simulink library "EntertainmentLevelDetectorBtc"  (R2022b)
settings: Solver=VariableStepAuto  StartTime=0.0  StopTime=10.0  RelTol=1e-3
libraries: TuneVar x25, LevelDetectorLibraryLib x4, PoolIirBtc x2, PooliirLib x2, HandyTextFile x1
settings Model: Creator=kl13806  LastModifiedBy=kl13806
settings SolverCC: AlgebraicLoopSolver=TrustRegion
settings DebuggingCC: UnconnectedInputMsg=warning  UnconnectedOutputMsg=warning  UnconnectedLineMsg=warning  SFMachineParentedDataDiag=warning
settings ModelReferenceCC: EnableRefExpFcnMdlSchedulingChecks=on
settings RTWCC: DLArmComputeVersion=19.05

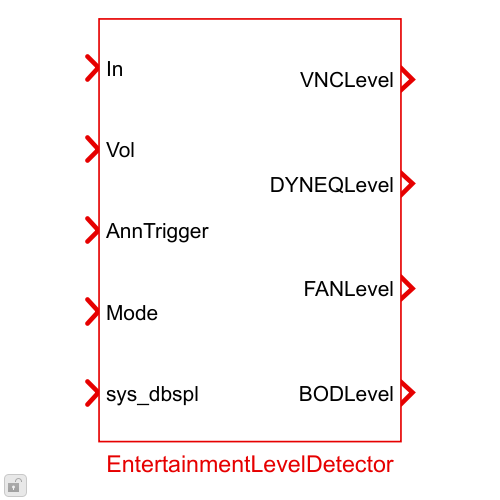
[thumbnail: Simulink's stored preview of the top-level diagram]
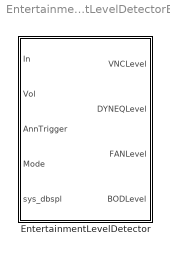
== system EntertainmentLevelDetectorBtc ==
  EntertainmentLevelDetector : Subsystem  mask(Level Detector for VNC, Dyanmic EQ, Fan and Boost-on-Demand){Config=[]}
      mask prompts: Config "EntertainmentLevelDetectorConfig"
      mask help: Level detector of entertainment audio in Audio Pilot.
      mask init:
      | blkh=gcbh;
      | Config=BTConfig.Assert(blkh,Config);
      | 
      | Config.Validate();

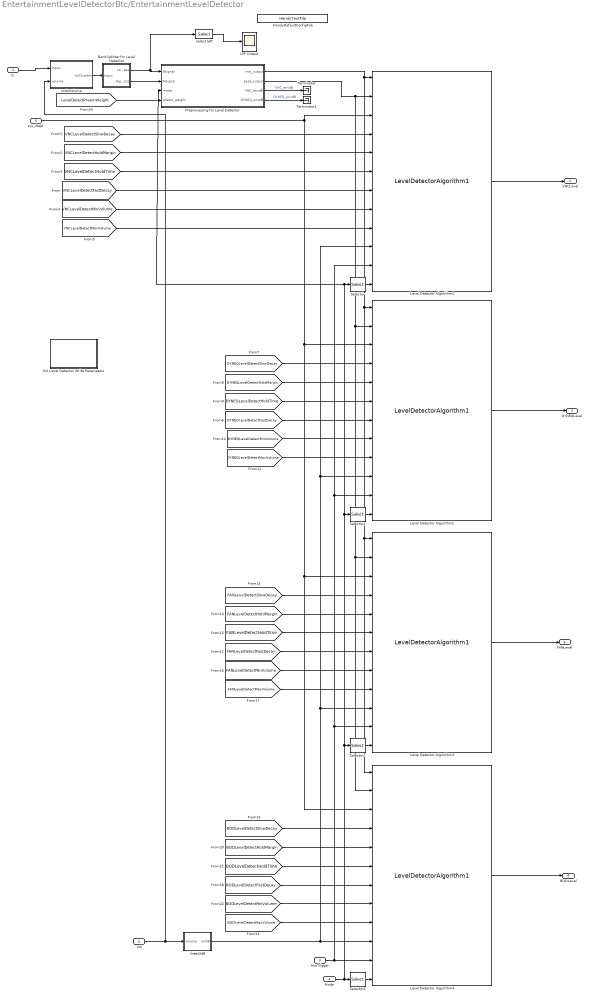
== system EntertainmentLevelDetectorBtc/EntertainmentLevelDetector ==
  In : Inport
  Vol : Inport  Port=2
  AnnTrigger : Inport  Port=3
  Mode : Inport  Port=4
  sys_dbspl : Inport  Port=5
  Band Splitter for Level Detector : Subsystem
  Ent Level Detector Write Parameters : Subsystem
  HandyDefaultConfigFile : HandyTextFile/HandyTextFile  TemplateSource=Config  FileSuffix=Init  OpenDialogOnLoad=off  UseThisBlockName=off  AddGrandParentNamePrefix=off  TheDefaultText=|  ShowInLibBrowser=on
      | % $(FILENAME) Setup model parameters for each "Init" callback (e.g. update diagram)
      | sample_rate_in_hertz = 44100;
      | frame_size = 32;
      | sysin_channel_count = 2;
      settings: SourceProductName=Bose Talaria
  LPF Output : Scope
  Level Detector Algorithm{1..4} (4 alike) : LevelDetectorLibraryLib/LevelDetectorAlgorithm1  Fd=Config.DlgDecRate
  Preprocessing for Level Detector : MATLAB Function  TreatAsAtomicUnit=on
  Selector : Selector  InputPortWidth=4  IndexOptions=Index vector (dialog)  Indices=[1]  OutputSizes=1
  Selector1 : Selector  InputPortWidth=4  IndexOptions=Index vector (dialog)  Indices=[2]  OutputSizes=1
  Selector2 : Selector  InputPortWidth=4  IndexOptions=Index vector (dialog)  Indices=[3]  OutputSizes=1
  Selector3 : Selector  InputPortWidth=4  IndexOptions=Index vector (dialog)  Indices=[4]  OutputSizes=1
  Terminator : Terminator
  Terminator1 : Terminator
  linear2dB : MATLAB Function  TreatAsAtomicUnit=on
  select left : Selector  NumberOfDimensions=2  InputPortWidth=3  IndexOptions=Select all,Index vector (dialog)  Indices=[1 3],1  OutputSizes=1,1
  undoVolume : MATLAB Function  TreatAsAtomicUnit=on
  VNCLevel : Outport  VectorParamsAs1DForOutWhenUnconnected=off
  DYNEQLevel : Outport  Port=2  VectorParamsAs1DForOutWhenUnconnected=off
  FANLevel : Outport  Port=3  VectorParamsAs1DForOutWhenUnconnected=off
  BODLevel : Outport  Port=4  VectorParamsAs1DForOutWhenUnconnected=off
  wires:
  In/1 -> undoVolume/1(input)
  undoVolume/1(fullScaleIn) -> Band Splitter for Level Detector/1(Input)
  [LevelDetectPreemWeight] -> Preprocessing for Level Detector/4(preem_weight)
  Preprocessing for Level Detector/4(DYNEQ_envdB) -> Terminator1/1  "DYNEQ_envdB"
  Preprocessing for Level Detector/3(VNC_envdB) -> Terminator/1  "VNC_envdB"
  [BODLevelDetectHoldMargin] -> Level Detector Algorithm4/5
  [BODLevelDetectHoldTime] -> Level Detector Algorithm4/6
  [BODLevelDetectSlowDecay] -> Level Detector Algorithm4/4
  [BODLevelDetectFastDecay] -> Level Detector Algorithm4/7
  Selector3/1 -> Level Detector Algorithm4/12
  Selector2/1 -> Level Detector Algorithm3/12
  Selector1/1 -> Level Detector Algorithm2/12
  Selector/1 -> Level Detector Algorithm1/12
  Mode/1 -> Selector/1, Preprocessing for Level Detector/3(mode), Selector1/1, Selector2/1, Selector3/1
  Level Detector Algorithm1/1 -> VNCLevel/1
  linear2dB/1(voldB) -> Level Detector Algorithm1/10, Level Detector Algorithm2/10, Level Detector Algorithm3/10, Level Detector Algorithm4/10
  sys_dbspl/1 -> Level Detector Algorithm1/3, Level Detector Algorithm3/3, Level Detector Algorithm4/3, Level Detector Algorithm2/3
  [VNCLevelDetectMaxVolume] -> Level Detector Algorithm1/9
  [BODLevelDetectMaxVolume] -> Level Detector Algorithm4/9
  [BODLevelDetectMinVolume] -> Level Detector Algorithm4/8
  Level Detector Algorithm4/1 -> BODLevel/1
  Preprocessing for Level Detector/2(peak_output) -> Level Detector Algorithm3/2, Level Detector Algorithm4/2, Level Detector Algorithm2/2, Level Detector Algorithm1/2
  [VNCLevelDetectMinVolume] -> Level Detector Algorithm1/8
  [VNCLevelDetectFastDecay] -> Level Detector Algorithm1/7
  [VNCLevelDetectHoldTime] -> Level Detector Algorithm1/6
  [VNCLevelDetectHoldMargin] -> Level Detector Algorithm1/5
  [VNCLevelDetectSlowDecay] -> Level Detector Algorithm1/4
  Vol/1 -> linear2dB/1(volume), undoVolume/2(volume)
  AnnTrigger/1 -> Level Detector Algorithm1/11, Level Detector Algorithm2/11, Level Detector Algorithm3/11, Level Detector Algorithm4/11
  select left/1 -> LPF Output/1
  [DYNEQLevelDetectSlowDecay] -> Level Detector Algorithm2/4
  [DYNEQLevelDetectHoldMargin] -> Level Detector Algorithm2/5
  [DYNEQLevelDetectHoldTime] -> Level Detector Algorithm2/6
  [DYNEQLevelDetectFastDecay] -> Level Detector Algorithm2/7
  [DYNEQLevelDetectMinVolume] -> Level Detector Algorithm2/8
  [DYNEQLevelDetectMaxVolume] -> Level Detector Algorithm2/9
  [FANLevelDetectSlowDecay] -> Level Detector Algorithm3/4
  [FANLevelDetectHoldMargin] -> Level Detector Algorithm3/5
  [FANLevelDetectHoldTime] -> Level Detector Algorithm3/6
  [FANLevelDetectFastDecay] -> Level Detector Algorithm3/7
  [FANLevelDetectMinVolume] -> Level Detector Algorithm3/8
  [FANLevelDetectMaxVolume] -> Level Detector Algorithm3/9
  Preprocessing for Level Detector/1(rms_output) -> Level Detector Algorithm3/1, Level Detector Algorithm4/1, Level Detector Algorithm2/1, Level Detector Algorithm1/1
  Band Splitter for Level Detector/1(LowPass) -> select left/1, Preprocessing for Level Detector/1(Bsignal)
  Band Splitter for Level Detector/2(HighPass) -> Preprocessing for Level Detector/2(Msignal)
  Level Detector Algorithm2/1 -> DYNEQLevel/1
  Level Detector Algorithm3/1 -> FANLevel/1

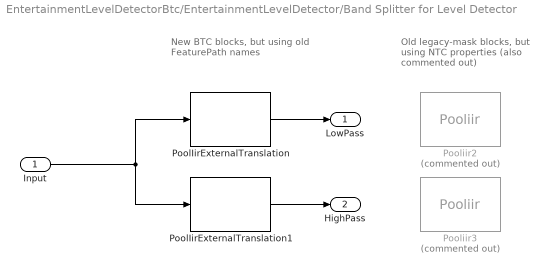
== system EntertainmentLevelDetectorBtc/EntertainmentLevelDetector/Band Splitter for Level Detector ==
  note: Old legacy-mask blocks,
      | but using NTC properties
      | (also commented out)
  note: New BTC blocks, but using
      | old FeaturePath names
  Input : Inport
  PoolIirExternalTranslation : PoolIirBtc/PoolIirExternalTranslation  Config=Config.level_detect_preemphasis_lpf_  FeatureName=level_detect_preemphasis_lpf_
      settings: SourceProductName=Bose Blocklib
  PoolIirExternalTranslation1 : PoolIirBtc/PoolIirExternalTranslation  Config=Config.level_detect_preemphasis_hpf_  FeatureName=level_detect_preemphasis_hpf_
      settings: SourceProductName=Bose Blocklib
  Pooliir2 : PooliirLib/Pooliir  Commented=on  maxNumStages=Config.DlgBsMaxNumStages  numStages=Config.DlgBsNumStages  coeffs=Config.DlgBsLpCoeffs  FeatureName=level_detect_preemphasis_lpf_
  Pooliir3 : PooliirLib/Pooliir  Commented=on  maxNumStages=Config.DlgBsMaxNumStages  numStages=Config.DlgBsNumStages  coeffs=Config.DlgBsHpCoeffs  FeatureName=level_detect_preemphasis_hpf_
  LowPass : Outport  VectorParamsAs1DForOutWhenUnconnected=off
  HighPass : Outport  Port=2  VectorParamsAs1DForOutWhenUnconnected=off
  wires:
  Input/1 -> PoolIirExternalTranslation1/1, PoolIirExternalTranslation/1
  PoolIirExternalTranslation/1 -> LowPass/1
  PoolIirExternalTranslation1/1 -> HighPass/1

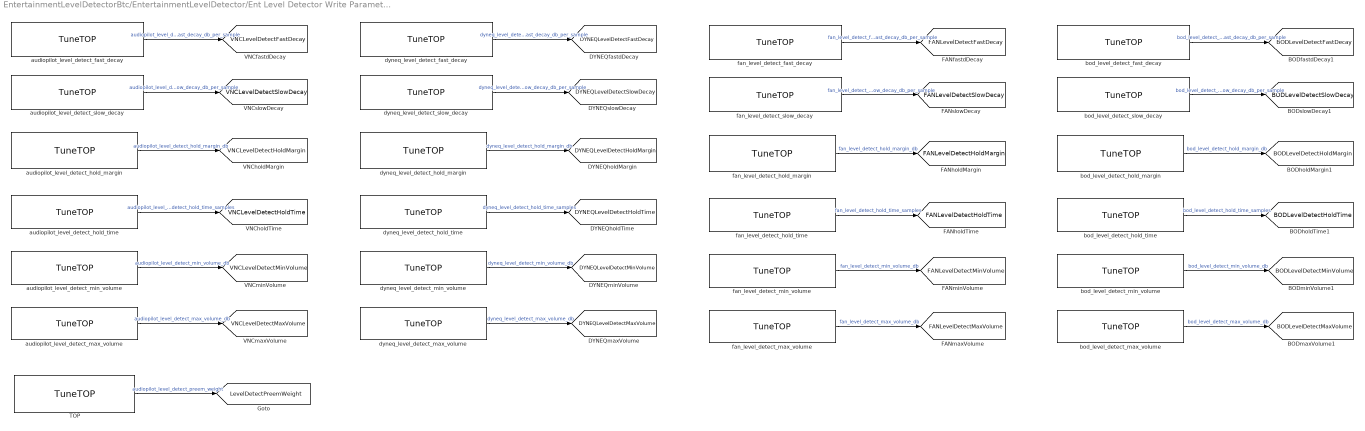
== system EntertainmentLevelDetectorBtc/EntertainmentLevelDetector/Ent Level Detector Write Parameters ==
  TOP : TuneVar/TuneTOP  TriggerInit=[-285 479 -80 541]  TopName=audiopilot_level_detect_preem_weight  TuneName=audiopilot_level_detect_preem_weight  DataType=Inherit: Same as input  TunabilityNumber=1  MinValue=[]  MaxValue=[]  BankNumber=0  PreOverlay=false  PostOverlay=false  UseSameName=on  MaskValue=single(4.0)
      settings: SourceProductName=Bose Talaria
  audiopilot_level_detect_fast_decay : TuneVar/TuneTOP  TriggerInit=[-290 -124 -65 -66]  TopName=audiopilot_level_detect_fast_decay_db_per_sample  TuneName=audiopilot_level_detect_fast_decay_db_per_sample  DataType=Inherit: Same as input  TunabilityNumber=1  MinValue=[]  MaxValue=[]  BankNumber=0  PreOverlay=false  PostOverlay=false  UseSameName=on  MaskValue=Config.DlgFastDecay
      settings: SourceProductName=Bose Talaria
  audiopilot_level_detect_hold_margin : TuneVar/TuneTOP  TriggerInit=[-290 64 -75 126]  TopName=audiopilot_level_detect_hold_margin_db  TuneName=audiopilot_level_detect_hold_margin_db  DataType=Inherit: Same as input  TunabilityNumber=1  MinValue=[]  MaxValue=[]  BankNumber=0  PreOverlay=false  PostOverlay=false  UseSameName=on  MaskValue=Config.DefaultHoldMargin
      settings: SourceProductName=Bose Talaria
  audiopilot_level_detect_hold_time : TuneVar/TuneTOP  TriggerInit=[-290 172 -75 228]  TopName=audiopilot_level_detect_hold_time_samples  TuneName=audiopilot_level_detect_hold_time_samples  DataType=Inherit: Same as input  TunabilityNumber=1  MinValue=[]  MaxValue=[]  BankNumber=0  PreOverlay=false  PostOverlay=false  UseSameName=on  MaskValue=Config.DlgHoldTime
      settings: SourceProductName=Bose Talaria
  audiopilot_level_detect_max_volume : TuneVar/TuneTOP  TriggerInit=[-290 362 -75 418]  TopName=audiopilot_level_detect_max_volume_db  TuneName=audiopilot_level_detect_max_volume_db  DataType=Inherit: Same as input  TunabilityNumber=1  MinValue=[]  MaxValue=[]  BankNumber=0  PreOverlay=false  PostOverlay=false  UseSameName=on  MaskValue=Config.DefaultMaxVolDbSpl
      settings: SourceProductName=Bose Talaria
  audiopilot_level_detect_min_volume : TuneVar/TuneTOP  TriggerInit=[-290 267 -75 323]  TopName=audiopilot_level_detect_min_volume_db  TuneName=audiopilot_level_detect_min_volume_db  DataType=Inherit: Same as input  TunabilityNumber=1  MinValue=[]  MaxValue=[]  BankNumber=0  PreOverlay=false  PostOverlay=false  UseSameName=on  MaskValue=Config.DefaultMinVolDpSpl
      settings: SourceProductName=Bose Talaria
  audiopilot_level_detect_slow_decay : TuneVar/TuneTOP  TriggerInit=[-290 -34 -65 24]  TopName=audiopilot_level_detect_slow_decay_db_per_sample  TuneName=audiopilot_level_detect_slow_decay_db_per_sample  DataType=Inherit: Same as input  TunabilityNumber=1  MinValue=[]  MaxValue=[]  BankNumber=0  PreOverlay=false  PostOverlay=false  UseSameName=on  MaskValue=Config.DlgSlowDecay
      settings: SourceProductName=Bose Talaria
  bod_level_detect_fast_decay : TuneVar/TuneTOP  TriggerInit=[1495 -119 1720 -61]  TopName=bod_level_detect_fast_decay_db_per_sample  TuneName=bod_level_detect_fast_decay_db_per_sample  DataType=Inherit: Same as input  TunabilityNumber=1  MinValue=[]  MaxValue=[]  BankNumber=0  PreOverlay=false  PostOverlay=false  UseSameName=on  MaskValue=Config.DlgFastDecay
      settings: SourceProductName=Bose Talaria
  bod_level_detect_hold_margin : TuneVar/TuneTOP  TriggerInit=[1495 69 1710 131]  TopName=bod_level_detect_hold_margin_db  TuneName=bod_level_detect_hold_margin_db  DataType=Inherit: Same as input  TunabilityNumber=1  MinValue=[]  MaxValue=[]  BankNumber=0  PreOverlay=false  PostOverlay=false  UseSameName=on  MaskValue=Config.DefaultHoldMargin
      settings: SourceProductName=Bose Talaria
  bod_level_detect_hold_time : TuneVar/TuneTOP  TriggerInit=[1495 177 1710 233]  TopName=bod_level_detect_hold_time_samples  TuneName=bod_level_detect_hold_time_samples  DataType=Inherit: Same as input  TunabilityNumber=1  MinValue=[]  MaxValue=[]  BankNumber=0  PreOverlay=false  PostOverlay=false  UseSameName=on  MaskValue=Config.DlgHoldTime
      settings: SourceProductName=Bose Talaria
  bod_level_detect_max_volume : TuneVar/TuneTOP  TriggerInit=[1495 367 1710 423]  TopName=bod_level_detect_max_volume_db  TuneName=bod_level_detect_max_volume_db  DataType=Inherit: Same as input  TunabilityNumber=1  MinValue=[]  MaxValue=[]  BankNumber=0  PreOverlay=false  PostOverlay=false  UseSameName=on  MaskValue=Config.DefaultMaxVolDbSpl
      settings: SourceProductName=Bose Talaria
  bod_level_detect_min_volume : TuneVar/TuneTOP  TriggerInit=[1495 272 1710 328]  TopName=bod_level_detect_min_volume_db  TuneName=bod_level_detect_min_volume_db  DataType=Inherit: Same as input  TunabilityNumber=1  MinValue=[]  MaxValue=[]  BankNumber=0  PreOverlay=false  PostOverlay=false  UseSameName=on  MaskValue=Config.DefaultMinVolDpSpl
      settings: SourceProductName=Bose Talaria
  bod_level_detect_slow_decay : TuneVar/TuneTOP  TriggerInit=[1495 -29 1720 29]  TopName=bod_level_detect_slow_decay_db_per_sample  TuneName=bod_level_detect_slow_decay_db_per_sample  DataType=Inherit: Same as input  TunabilityNumber=1  MinValue=[]  MaxValue=[]  BankNumber=0  PreOverlay=false  PostOverlay=false  UseSameName=on  MaskValue=Config.DlgSlowDecay
      settings: SourceProductName=Bose Talaria
  dyneq_level_detect_fast_decay : TuneVar/TuneTOP  TriggerInit=[305 -124 530 -66]  TopName=dyneq_level_detect_fast_decay_db_per_sample  TuneName=dyneq_level_detect_fast_decay_db_per_sample  DataType=Inherit: Same as input  TunabilityNumber=1  MinValue=[]  MaxValue=[]  BankNumber=0  PreOverlay=false  PostOverlay=false  UseSameName=on  MaskValue=Config.DlgFastDecay
      settings: SourceProductName=Bose Talaria
  dyneq_level_detect_hold_margin : TuneVar/TuneTOP  TriggerInit=[305 64 520 126]  TopName=dyneq_level_detect_hold_margin_db  TuneName=dyneq_level_detect_hold_margin_db  DataType=Inherit: Same as input  TunabilityNumber=1  MinValue=[]  MaxValue=[]  BankNumber=0  PreOverlay=false  PostOverlay=false  UseSameName=on  MaskValue=Config.DefaultHoldMargin
      settings: SourceProductName=Bose Talaria
  dyneq_level_detect_hold_time : TuneVar/TuneTOP  TriggerInit=[305 172 520 228]  TopName=dyneq_level_detect_hold_time_samples  TuneName=dyneq_level_detect_hold_time_samples  DataType=Inherit: Same as input  TunabilityNumber=1  MinValue=[]  MaxValue=[]  BankNumber=0  PreOverlay=false  PostOverlay=false  UseSameName=on  MaskValue=Config.DlgHoldTime
      settings: SourceProductName=Bose Talaria
  dyneq_level_detect_max_volume : TuneVar/TuneTOP  TriggerInit=[305 362 520 418]  TopName=dyneq_level_detect_max_volume_db  TuneName=dyneq_level_detect_max_volume_db  DataType=Inherit: Same as input  TunabilityNumber=1  MinValue=[]  MaxValue=[]  BankNumber=0  PreOverlay=false  PostOverlay=false  UseSameName=on  MaskValue=Config.DefaultMaxVolDbSpl
      settings: SourceProductName=Bose Talaria
  dyneq_level_detect_min_volume : TuneVar/TuneTOP  TriggerInit=[305 267 520 323]  TopName=dyneq_level_detect_min_volume_db  TuneName=dyneq_level_detect_min_volume_db  DataType=Inherit: Same as input  TunabilityNumber=1  MinValue=[]  MaxValue=[]  BankNumber=0  PreOverlay=false  PostOverlay=false  UseSameName=on  MaskValue=Config.DefaultMinVolDpSpl
      settings: SourceProductName=Bose Talaria
  dyneq_level_detect_slow_decay : TuneVar/TuneTOP  TriggerInit=[305 -34 530 24]  TopName=dyneq_level_detect_slow_decay_db_per_sample  TuneName=dyneq_level_detect_slow_decay_db_per_sample  DataType=Inherit: Same as input  TunabilityNumber=1  MinValue=[]  MaxValue=[]  BankNumber=0  PreOverlay=false  PostOverlay=false  UseSameName=on  MaskValue=Config.DlgSlowDecay
      settings: SourceProductName=Bose Talaria
  fan_level_detect_fast_decay : TuneVar/TuneTOP  TriggerInit=[900 -119 1125 -61]  TopName=fan_level_detect_fast_decay_db_per_sample  TuneName=fan_level_detect_fast_decay_db_per_sample  DataType=Inherit: Same as input  TunabilityNumber=1  MinValue=[]  MaxValue=[]  BankNumber=0  PreOverlay=false  PostOverlay=false  UseSameName=on  MaskValue=Config.DlgFastDecay
      settings: SourceProductName=Bose Talaria
  fan_level_detect_hold_margin : TuneVar/TuneTOP  TriggerInit=[900 69 1115 131]  TopName=fan_level_detect_hold_margin_db  TuneName=fan_level_detect_hold_margin_db  DataType=Inherit: Same as input  TunabilityNumber=1  MinValue=[]  MaxValue=[]  BankNumber=0  PreOverlay=false  PostOverlay=false  UseSameName=on  MaskValue=Config.DefaultHoldMargin
      settings: SourceProductName=Bose Talaria
  fan_level_detect_hold_time : TuneVar/TuneTOP  TriggerInit=[900 177 1115 233]  TopName=fan_level_detect_hold_time_samples  TuneName=fan_level_detect_hold_time_samples  DataType=Inherit: Same as input  TunabilityNumber=1  MinValue=[]  MaxValue=[]  BankNumber=0  PreOverlay=false  PostOverlay=false  UseSameName=on  MaskValue=Config.DlgHoldTime
      settings: SourceProductName=Bose Talaria
  fan_level_detect_max_volume : TuneVar/TuneTOP  TriggerInit=[900 367 1115 423]  TopName=fan_level_detect_max_volume_db  TuneName=fan_level_detect_max_volume_db  DataType=Inherit: Same as input  TunabilityNumber=1  MinValue=[]  MaxValue=[]  BankNumber=0  PreOverlay=false  PostOverlay=false  UseSameName=on  MaskValue=Config.DefaultMaxVolDbSpl
      settings: SourceProductName=Bose Talaria
  fan_level_detect_min_volume : TuneVar/TuneTOP  TriggerInit=[900 272 1115 328]  TopName=fan_level_detect_min_volume_db  TuneName=fan_level_detect_min_volume_db  DataType=Inherit: Same as input  TunabilityNumber=1  MinValue=[]  MaxValue=[]  BankNumber=0  PreOverlay=false  PostOverlay=false  UseSameName=on  MaskValue=Config.DefaultMinVolDpSpl
      settings: SourceProductName=Bose Talaria
  fan_level_detect_slow_decay : TuneVar/TuneTOP  TriggerInit=[900 -29 1125 29]  TopName=fan_level_detect_slow_decay_db_per_sample  TuneName=fan_level_detect_slow_decay_db_per_sample  DataType=Inherit: Same as input  TunabilityNumber=1  MinValue=[]  MaxValue=[]  BankNumber=0  PreOverlay=false  PostOverlay=false  UseSameName=on  MaskValue=Config.DlgSlowDecay
      settings: SourceProductName=Bose Talaria
  tag scope: BODLevelDetectFastDecay=global, BODLevelDetectHoldMargin=global, BODLevelDetectHoldTime=global, BODLevelDetectMaxVolume=global, BODLevelDetectMinVolume=global, BODLevelDetectSlowDecay=global, DYNEQLevelDetectFastDecay=global, DYNEQLevelDetectHoldMargin=global, DYNEQLevelDetectHoldTime=global, DYNEQLevelDetectMaxVolume=global, DYNEQLevelDetectMinVolume=global, DYNEQLevelDetectSlowDecay=global, FANLevelDetectFastDecay=global, FANLevelDetectHoldMargin=global, FANLevelDetectHoldTime=global, FANLevelDetectMaxVolume=global, FANLevelDetectMinVolume=global, FANLevelDetectSlowDecay=global, LevelDetectPreemWeight=global, VNCLevelDetectFastDecay=global, VNCLevelDetectHoldMargin=global, VNCLevelDetectHoldTime=global, VNCLevelDetectMaxVolume=global, VNCLevelDetectMinVolume=global, VNCLevelDetectSlowDecay=global
  wires:
  TOP/1 -> [LevelDetectPreemWeight]  "audiopilot_level_detect_preem_weight"
  bod_level_detect_max_volume/1 -> [BODLevelDetectMaxVolume]  "bod_level_detect_max_volume_db"
  bod_level_detect_min_volume/1 -> [BODLevelDetectMinVolume]  "bod_level_detect_min_volume_db"
  bod_level_detect_hold_time/1 -> [BODLevelDetectHoldTime]  "bod_level_detect_hold_time_samples"
  bod_level_detect_hold_margin/1 -> [BODLevelDetectHoldMargin]  "bod_level_detect_hold_margin_db"
  bod_level_detect_slow_decay/1 -> [BODLevelDetectSlowDecay]  "bod_level_detect_slow_decay_db_per_sample"
  bod_level_detect_fast_decay/1 -> [BODLevelDetectFastDecay]  "bod_level_detect_fast_decay_db_per_sample"
  fan_level_detect_max_volume/1 -> [FANLevelDetectMaxVolume]  "fan_level_detect_max_volume_db"
  fan_level_detect_min_volume/1 -> [FANLevelDetectMinVolume]  "fan_level_detect_min_volume_db"
  fan_level_detect_hold_time/1 -> [FANLevelDetectHoldTime]  "fan_level_detect_hold_time_samples"
  fan_level_detect_hold_margin/1 -> [FANLevelDetectHoldMargin]  "fan_level_detect_hold_margin_db"
  fan_level_detect_slow_decay/1 -> [FANLevelDetectSlowDecay]  "fan_level_detect_slow_decay_db_per_sample"
  fan_level_detect_fast_decay/1 -> [FANLevelDetectFastDecay]  "fan_level_detect_fast_decay_db_per_sample"
  dyneq_level_detect_max_volume/1 -> [DYNEQLevelDetectMaxVolume]  "dyneq_level_detect_max_volume_db"
  dyneq_level_detect_min_volume/1 -> [DYNEQLevelDetectMinVolume]  "dyneq_level_detect_min_volume_db"
  dyneq_level_detect_hold_time/1 -> [DYNEQLevelDetectHoldTime]  "dyneq_level_detect_hold_time_samples"
  dyneq_level_detect_hold_margin/1 -> [DYNEQLevelDetectHoldMargin]  "dyneq_level_detect_hold_margin_db"
  dyneq_level_detect_slow_decay/1 -> [DYNEQLevelDetectSlowDecay]  "dyneq_level_detect_slow_decay_db_per_sample"
  dyneq_level_detect_fast_decay/1 -> [DYNEQLevelDetectFastDecay]  "dyneq_level_detect_fast_decay_db_per_sample"
  audiopilot_level_detect_max_volume/1 -> [VNCLevelDetectMaxVolume]  "audiopilot_level_detect_max_volume_db"
  audiopilot_level_detect_min_volume/1 -> [VNCLevelDetectMinVolume]  "audiopilot_level_detect_min_volume_db"
  audiopilot_level_detect_hold_time/1 -> [VNCLevelDetectHoldTime]  "audiopilot_level_detect_hold_time_samples"
  audiopilot_level_detect_hold_margin/1 -> [VNCLevelDetectHoldMargin]  "audiopilot_level_detect_hold_margin_db"
  audiopilot_level_detect_slow_decay/1 -> [VNCLevelDetectSlowDecay]  "audiopilot_level_detect_slow_decay_db_per_sample"
  audiopilot_level_detect_fast_decay/1 -> [VNCLevelDetectFastDecay]  "audiopilot_level_detect_fast_decay_db_per_sample"

== matlab function EntertainmentLevelDetectorBtc/EntertainmentLevelDetector/Preprocessing for Level Detector ==
  data: Bsignal input; Msignal input; rms_output output; mode input; peak_output output; VNC_envdB output; DYNEQ_envdB output; preem_weight input
function [rms_output, peak_output, VNC_envdB, DYNEQ_envdB] = preprocessWithPreemphasis(Bsignal, Msignal, mode, preem_weight)
% Initialize RMS_MODE
RMS_MODE = single(1.0);
% Initialize modePeak
modePeak = sum(mode > RMS_MODE);
% Initialize weight
weight = preem_weight; %mid range weight vs bass
% Computing currB
currB = 10 * log10(max(mean(Bsignal .* Bsignal, 1)) + eps);
% Computing currB
currM = 10 * log10(max(mean(Msignal .* Msignal, 1)) + eps);
% Computing rms_output
rms_output = max(currB, currM + weight);
% Check whetjer modepeak is greater than zero and compute currB, currM &
% peak_output
if (modePeak > 0)
    currB = 20 * log10(max(max(abs(Bsignal))) + eps);
    currM = 20 * log10(max(max(abs(Msignal))) + eps);
    peak_output = max(currB, currM + weight);
else
    % if not compute peak_output as rms_output
    peak_output = rms_output;
end
% Check if mode(1) is greater than RMS_MODE and compute VNC_envdB
if (mode(1) > RMS_MODE)
    VNC_envdB = peak_output;
else
    % If not compute VNC_envdB as rms_output
    VNC_envdB = rms_output;
end
% Check if mode(2) is greater than RMS_MODE and compute DYNEQ_envdB
if (mode(2) > RMS_MODE)
    DYNEQ_envdB = peak_output;
else
    % If not compute DYNEQ_envdB as rms_output
    DYNEQ_envdB = rms_output;
end

== matlab function EntertainmentLevelDetectorBtc/EntertainmentLevelDetector/undoVolume ==
  data: input input; volume input; fullScaleIn output
function fullScaleIn = fcn(input, volume)
% Initialize the parameters
fullScaleIn = single(input/(volume + eps));

== matlab function EntertainmentLevelDetectorBtc/EntertainmentLevelDetector/linear2dB ==
  data: volume input; voldB output
function voldB = fcn(volume)
% Compute voldB
voldB = single(20 * log10(volume + eps));
